simulink model "sampleModel27"  (R2021a)
settings: Solver=VariableStepAuto  StartTime=0.0  StopTime=10.0  RelTol=1e-3
undefined symbols (not defined in the file): DiscIntNeverNeededParam, magnitude, Newton, Raphson
libraries: simulink x49, pid_lib x7
(part 1 of 2)
settings Model: SimulationMode=accelerator  Creator=user  LastModifiedBy=CMelt

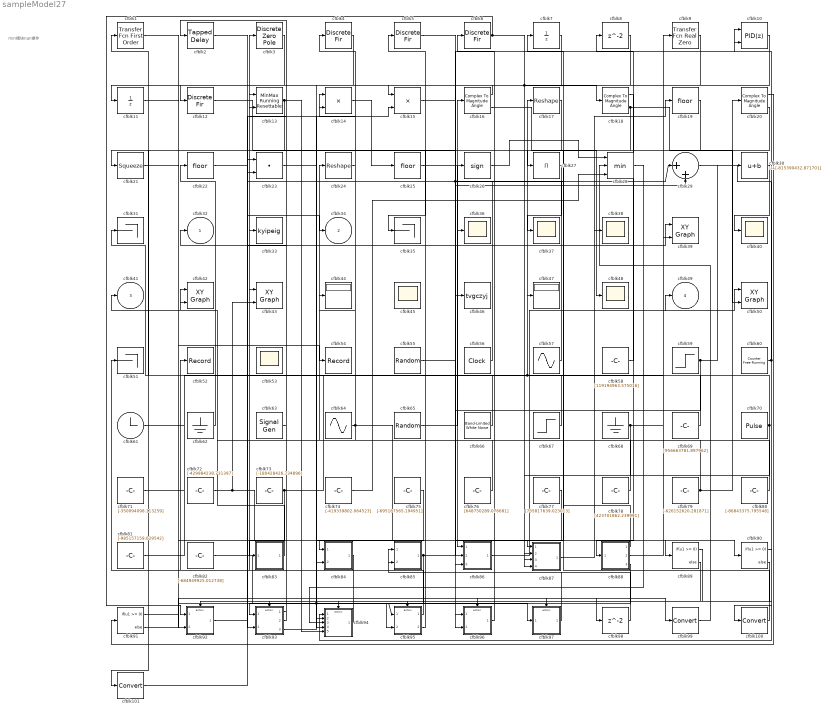
== system sampleModel27 ==
  note: min模块nan操作
  cfblk1 : simulink/Discrete/Transfer Fcn First Order  PoleZ=0.95  ICPrevOutput=0.0  DoSatur=off
  cfblk10 : pid_lib/PID Controller (2DOF)  Controller=PID  Form=Parallel  TimeDomain=Discrete-time  UseExternalTs=off  SampleTime=1  IntegratorMethod=Forward Euler  FilterMethod=Forward Euler  ControllerParametersSource=internal  P=1  I=1  D=0  UseFilter=on  N=100  b=1  c=1  TunerSelectOption=Transfer Function Based (PID Tuner App)  InitialConditionSource=internal  InitialConditionForIntegrator=0  InitialConditionForFilter=0  DifferentiatorICPrevScaledInput=0  ExternalReset=none  TrackingMode=off  Kt=1  LimitOutput=off  SatLimitsSource=internal  UpperSaturationLimit=inf  LowerSaturationLimit=-inf  LinearizeAsGain=off  AntiWindupMode=none  Kb=1  POutMin=[]  POutMax=[]  IOutMin=[]  IOutMax=[]  DOutMin=[]  DOutMax=[]  NOutMin=[]  NOutMax=[]  bOutMin=[]  bOutMax=[]  cOutMin=[]  cOutMax=[]  SumOutMin=[]  SumOutMax=[]  SaturationOutMin=[]  SaturationOutMax=[]  PParamMin=[]  PParamMax=[]  IParamMin=[]  IParamMax=[]  DParamMin=[]  DParamMax=[]  NParamMin=[]  NParamMax=[]  bParamMin=[]  bParamMax=[]  cParamMin=[]  cParamMax=[]  KbParamMin=[]  KbParamMax=[]  KtParamMin=[]  KtParamMax=[]  KbOutMin=[]  KbOutMax=[]  KtOutMin=[]  KtOutMax=[]  IntegratorOutMin=[]  IntegratorOutMax=[]  FilterOutMin=[]  FilterOutMax=[]  SumI1OutMin=[]  SumI1OutMax=[]  SumI2OutMin=[]  SumI2OutMax=[]  SumI3OutMin=[]  SumI3OutMax=[]  SumI4OutMin=[]  SumI4OutMax=[]  SumDOutMin=[]  SumDOutMax=[]  Sum1OutMin=[]  Sum1OutMax=[]  Sum2OutMin=[]  Sum2OutMax=[]  Sum3OutMin=[]  Sum3OutMax=[]  DifferentiatorOutMin=[]  DifferentiatorOutMax=[]  FilterDiffOutCoefMin=[]  FilterDiffOutCoefMax=[]  ReciprocalOutMin=[]  ReciprocalOutMax=[]  SumDenOutMin=[]  SumDenOutMax=[]  SumNumOutMin=[]  SumNumOutMax=[]  DivideOutMin=[]  DivideOutMax=[]  UdiffTsProdOutMin=[]  UdiffTsProdOutMax=[]  NTsProdOutMin=[]  NTsProdOutMax=[]  UintegralTsProdOutMin=[]  UintegralTsProdOutMax=[]  UngainTsProdOutMin=[]  UngainTsProdOutMax=[]  IntegratorContinuousStateAttributes=''  IntegratorStateMustResolveToSignalObject=off  IntegratorRTWStateStorageClass=Auto  FilterContinuousStateAttributes=''  FilterStateMustResolveToSignalObject=off  FilterRTWStateStorageClass=Auto  ParallelPVariant=InternalParameters  IdealPVariant=Disabled  IVariant=InternalParameters  DVariant=InternalParameters  bVariant=InternalParameters  cVariant=InternalParameters  IntegratorVariant=Discrete  SatVariant=Disabled  AWVariant=Passthrough  PCopyVariant=Disabled  TRVariant=Disabled  FdbkBlocksVariant=Forward  IdealPFdbkVariant=Disabled  SatFdbkVariant=Disabled  DerivativeFilterVariant=ForwardEulerFilter  NVariant=InternalParameters  NCopyVariant=Disabled  FilterICVariant=InternalICsFilter  IntegratorICVariant=InternalICs  ExternalResetVariant=Disabled  TRSumVariant=Passthrough  SumFdbkVariant=Disabled  SumVariant=Sum_PID  TsampFilterVariant=InternalTs  TsampNgainVariant=Passthrough  TsampIntegralVariant=Passthrough  ExternalSaturationOutDataTypeStr=Inherit: Same as second input
      settings: SourceProductBaseCode=SL
  cfblk100 : DataTypeConversion
  cfblk101 : DataTypeConversion
  cfblk11 : UnitDelay  HasFrameUpgradeWarning=on
  cfblk{4..6,12} (4 alike) : DiscreteFir  SampleTime=1
  cfblk13 : simulink/Math Operations/MinMax Running Resettable  Function=min  vinit=0.0
  cfblk14 : Product  Inputs=**
  cfblk15 : Product  Inputs=**
  cfblk16 : ComplexToMagnitudeAngle
  cfblk17 : Reshape
  cfblk18 : ComplexToMagnitudeAngle
  cfblk19 : Rounding
  cfblk2 : simulink/Discrete/Tapped Delay  vinit=0.0  samptime=-1  NumDelays=1  DelayOrder=Oldest  includeCurrent=off
  cfblk20 : ComplexToMagnitudeAngle
  cfblk21 : Squeeze
  cfblk22 : Rounding
  cfblk23 : DotProduct  InputSameDT=on  OutDataTypeStr=Inherit: Inherit via internal rule
  cfblk24 : Reshape
  cfblk25 : Rounding
  cfblk26 : Signum
  cfblk27 : Product  Inputs=*
  cfblk28 : MinMax  Inputs=3
  cfblk29 : Sum  Inputs=|++
  cfblk3 : DiscreteZeroPole  Poles=[0 0.5]  Gain=1
  cfblk30 : Bias  Bias=[-815390432.871701]
  cfblk31 : Terminator
  cfblk33 : ToWorkspace  VariableName=kyipeig  SaveFormat=Timeseries  SampleTime=-1
  cfblk35 : Terminator
  cfblk{36..38,40,45,48,53} (7 alike) : Scope
      cfblk45 settings: Floating=on
      cfblk53 settings: Floating=on
  cfblk{39,42..43,50} (4 alike) : simulink/Sinks/XY Graph  xmin=-1  xmax=1  ymin=-1  ymax=1  st=-1
  cfblk44 : Display
  cfblk46 : ToWorkspace  VariableName=tvgczyj  SaveFormat=Timeseries  SampleTime=-1
  cfblk47 : Display
  cfblk51 : Terminator
  cfblk52 : Record  FileSettingsInternal="{\"entries\":[{\"content\":{\"excelSettings\":{\"content\":{},\"type\":\"Streamout.ExcelSettings\"}},\"type\":\"Streamout.FileSettingStorage\",\"uuid\":\"fb11f80e-34bd-4155-aeb7-01b810d6d789\"}],\"packageUris\":[\"http://schema.mathworks.com/mf0/streamout_blocks/R2020a\"],\"version\":\"1.0\"}"  SignalsInternal="{\"entries\":[{\"content\":{\"signals\":[{\"content\":{\"blockPath\":[\"sampleModel27/cfblk52\"],\"channel\":[],\"dimensions\":[1],\"domain\":\"samplemodel27/cfblk52\",\"lineColor\":\"#a2142f\",\"plots\":[1],\"port\":1,\"sid\":[\"\"],\"signalID\":891,\"signalName\":\"cfblk84\"},\"type\":\"RecordBlkView.Signal\",\"uuid\":\"6f85a095-4475-43d3-bab9-3dbcc0fecad7\"}]},\"type\":\"RecordBlkView.InputSignals\",\"uuid\":\"24e3b0c2-4f19-493b-93a7-05a205e117ae\"}],\"packageUris\":[\"http://schema.mathworks.com/mf0/streamout_blocks/R2020a\"],\"version\":\"1.0\"}"  VisualizationBindings="{\"sparklinesplugin\":{\"info\":[{\"bindingParametersList\":[],\"subplotID\":1}]}}"
  cfblk54 : Record  FileSettingsInternal="{\"entries\":[{\"content\":{\"excelSettings\":{\"content\":{},\"type\":\"Streamout.ExcelSettings\"}},\"type\":\"Streamout.FileSettingStorage\",\"uuid\":\"661a3fc6-d036-46d0-a4c7-a8be5b92de13\"}],\"packageUris\":[\"http://schema.mathworks.com/mf0/streamout_blocks/R2020a\"],\"version\":\"1.0\"}"  SignalsInternal="{\"entries\":[{\"content\":{\"signals\":[{\"content\":{\"blockPath\":[\"sampleModel27/cfblk54\"],\"channel\":[],\"dimensions\":[1],\"domain\":\"samplemodel27/cfblk54\",\"lineColor\":\"#139fff\",\"plots\":[1],\"port\":1,\"sid\":[\"\"],\"signalID\":895,\"signalName\":\"cfblk21\"},\"type\":\"RecordBlkView.Signal\",\"uuid\":\"1e160afe-88b1-4798-9b6e-19891c68b1a2\"}]},\"type\":\"RecordBlkView.InputSignals\",\"uuid\":\"bd873b34-5c71-4cc0-af38-2544e9a0ace2\"}],\"packageUris\":[\"http://schema.mathworks.com/mf0/streamout_blocks/R2020a\"],\"version\":\"1.0\"}"  VisualizationBindings="{\"sparklinesplugin\":{\"info\":[{\"bindingParametersList\":[],\"subplotID\":1}]}}"
  cfblk55 : RandomNumber  Mean=[-1249.450853]  Variance=[75448.037597]  Seed=[754077994.000000]  SampleTime=0.1
  cfblk56 : DigitalClock
  cfblk57 : Sin  Amplitude=[-963722435.247906]  Bias=[930160760.058033]  SampleTime=0
  cfblk58 : Constant  Value=[119194963.575016]  SampleTime=1
  cfblk59 : Step  Time=[33.000000]  Before=[-955328328.233696]  After=[-779935419.294909]  SampleTime=0
  cfblk60 : simulink/Sources/Counter Free-Running  NumBits=[42.000000]  tsamp=-1
  cfblk61 : Clock
  cfblk62 : Ground
  cfblk63 : SignalGenerator  WaveForm=sawtooth  Amplitude=[910247910.621120]  Units=rad/sec
  cfblk64 : Sin  Amplitude=[-129917709.975789]  Bias=[-276116717.461174]  SampleTime=0
  cfblk65 : UniformRandomNumber  Minimum=[-3659398183.640169]  Maximum=[7187088124.881099]  Seed=[85361646.000000]  SampleTime=0.1
  cfblk66 : simulink/Sources/Band-Limited White Noise  Cov=[7101691506.405921]  Ts=0.1  seed=[513787139.000000]
  cfblk67 : Step  Time=[17.000000]  Before=[136149007.270913]  After=[-603107143.045370]  SampleTime=0
  cfblk68 : Ground
  cfblk69 : Constant  Value=[956663781.897962]  SampleTime=1
  cfblk7 : UnitDelay  HasFrameUpgradeWarning=on
  cfblk70 : DiscretePulseGenerator  PulseType=Time based  Amplitude=[-722737795.690040]  Period=[17925385.343940]  PulseWidth=5  PhaseDelay=[6.000000]
  cfblk71 : Constant  Value=[-350094098.113259]  SampleTime=1
  cfblk72 : Constant  Value=[-429984238.731397]  SampleTime=1
  cfblk73 : Constant  Value=[-180428426.734896]  SampleTime=1
  cfblk74 : Constant  Value=[-419339802.064523]  SampleTime=1
  cfblk75 : Constant  Value=[-695187565.194951]  SampleTime=1
  cfblk76 : Constant  Value=[648750289.076681]  SampleTime=1
  cfblk77 : Constant  Value=[735817639.023013]  SampleTime=1
  cfblk78 : Constant  Value=[423701862.239991]  SampleTime=1
  cfblk79 : Constant  Value=[-626152620.281871]  SampleTime=1
  cfblk8 : Delay  SampleTime=1
  cfblk80 : Constant  Value=[-86843375.795548]  SampleTime=1
  cfblk81 : Constant  Value=[-985157159.629542]  SampleTime=1
  cfblk82 : Constant  Value=[-684949925.012738]  SampleTime=1
  cfblk83 : Subsystem
  cfblk84 : Subsystem
  cfblk85 : Subsystem
  cfblk86 : Subsystem
  cfblk87 : Subsystem
  cfblk88 : Subsystem
  cfblk89 : If  IfExpression=u1 >= 0  SampleTime=1
  cfblk9 : simulink/Discrete/Transfer Fcn Real Zero  ZeroZ=0.75  ICPrevInput=0.0  DoSatur=off
      settings: SourceProductBaseCode=SL
  cfblk90 : If  IfExpression=u1 >= 0  SampleTime=1
  cfblk91 : If  IfExpression=u1 >= 0  SampleTime=1
  cfblk92 : Subsystem  TreatAsAtomicUnit=on
  cfblk93 : Subsystem  TreatAsAtomicUnit=on
  cfblk94 : Subsystem  TreatAsAtomicUnit=on
  cfblk95 : Subsystem  TreatAsAtomicUnit=on
  cfblk96 : Subsystem  TreatAsAtomicUnit=on
  cfblk97 : Subsystem  TreatAsAtomicUnit=on
  cfblk98 : Delay  SampleTime=1
  cfblk99 : DataTypeConversion
  cfblk32 : Outport
  cfblk34 : Outport  Port=2
  cfblk41 : Outport  Port=3
  cfblk49 : Outport  Port=4
  wires:
  cfblk3/1 -> cfblk11/1
  cfblk56/1 -> cfblk2/1
  cfblk57/1 -> cfblk6/1
  cfblk65/1 -> cfblk16/1
  cfblk72/1 -> cfblk89/1, cfblk43/2
  cfblk84/1(cfblk2) -> cfblk52/1
  cfblk6/1 -> cfblk92/1(cfblk1), cfblk18/1
  cfblk61/1 -> cfblk17/1
  cfblk94/1(cfblk2) -> cfblk3/1
  cfblk76/1 -> cfblk24/1
  cfblk64/1 -> cfblk14/1, cfblk90/1
  cfblk97/1(cfblk2) -> cfblk85/1(cfblk1)
  cfblk25/1 -> cfblk86/1(cfblk1)
  cfblk60/1 -> cfblk10/1, cfblk100/1
  cfblk19/1 -> cfblk27/1
  cfblk88/1(cfblk2) -> cfblk7/1
  cfblk22/1 -> cfblk14/2
  cfblk86/1(cfblk2) -> cfblk49/1
  cfblk70/1 -> cfblk36/1, cfblk87/2(cfblk11)
  cfblk55/1 -> cfblk96/1(cfblk1)
  cfblk96/1(cfblk2) -> cfblk26/1
  cfblk10/1 -> cfblk86/2(cfblk9), cfblk87/4(cfblk13)
  cfblk16/1 -> cfblk15/1
  cfblk62/1 -> cfblk41/1
  cfblk88/2(cfblk9) -> cfblk50/1
  cfblk16/2 -> cfblk48/1
  cfblk85/1(cfblk2) -> cfblk29/1, cfblk10/2, cfblk95/2(cfblk13)
  cfblk2/1 -> cfblk34/1
  cfblk4/1 -> cfblk92/2(cfblk11)
  cfblk29/1 -> cfblk94/1(cfblk1)
  cfblk26/1 -> cfblk28/1
  cfblk67/1 -> cfblk1/1
  cfblk1/1 -> cfblk97/1(cfblk1)
  cfblk63/1 -> cfblk13/1
  cfblk66/1 -> cfblk22/1
  cfblk71/1 -> cfblk9/1
  cfblk14/1 -> cfblk25/1
  cfblk21/1 -> cfblk54/1
  cfblk24/1 -> cfblk4/1
  cfblk95/1(cfblk2) -> cfblk51/1
  cfblk12/1 -> cfblk46/1
  cfblk81/1 -> cfblk33/1
  cfblk17/1 -> cfblk35/1
  cfblk18/1 -> cfblk88/1(cfblk1)
  cfblk88/3(cfblk10) -> cfblk93/1(cfblk1)
  cfblk77/1 -> cfblk96/2(cfblk7)
  cfblk75/1 -> cfblk94/2(cfblk13)
  cfblk9/1 -> cfblk12/1
  cfblk83/1(cfblk2) -> cfblk42/1
  cfblk95/2(cfblk14) -> cfblk5/1
  cfblk80/1 -> cfblk44/1
  cfblk7/1 -> cfblk93/2(cfblk13)
  cfblk11/1 -> cfblk84/1(cfblk1)
  cfblk58/1 -> cfblk8/1
  cfblk18/2 -> cfblk50/2, cfblk87/1(cfblk1)
  cfblk27/1 -> cfblk37/1
  cfblk69/1 -> cfblk47/1, cfblk31/1
  cfblk15/1 -> cfblk29/2
  cfblk8/1 -> cfblk84/2(cfblk9)
  cfblk82/1 -> cfblk95/1(cfblk1), cfblk94/4(cfblk15)
  cfblk13/1 -> cfblk94/5(cfblk16), cfblk101/1
  cfblk30/1 -> cfblk40/1
  cfblk20/1 -> cfblk91/1
  cfblk28/1 -> cfblk94/3(cfblk14)
  cfblk73/1 -> cfblk38/1, cfblk83/1(cfblk1)
  cfblk79/1 -> cfblk20/1, cfblk42/2
  cfblk93/1(cfblk2) -> cfblk13/2
  cfblk20/2 -> cfblk21/1
  cfblk92/1(cfblk2) -> cfblk39/1
  cfblk59/1 -> cfblk86/3(cfblk10), cfblk30/1
  cfblk93/2(cfblk14) -> cfblk32/1
  cfblk68/1 -> cfblk39/2, cfblk87/3(cfblk12)
  cfblk74/1 -> cfblk28/3
  cfblk78/1 -> cfblk43/1
  cfblk93/3(cfblk15) -> cfblk15/2
  cfblk87/1(cfblk2) -> cfblk19/1
  cfblk89/1 -> cfblk92/Action
  cfblk89/2 -> cfblk93/Action
  cfblk90/1 -> cfblk94/Action
  cfblk90/2 -> cfblk95/Action
  cfblk91/1 -> cfblk96/Action
  cfblk91/2 -> cfblk97/Action
  cfblk5/1 -> cfblk98/1
  cfblk98/1 -> cfblk85/2(cfblk14)
  cfblk23/1 -> cfblk99/1
  cfblk99/1 -> cfblk28/2
  cfblk100/1 -> cfblk23/1
  cfblk101/1 -> cfblk23/2

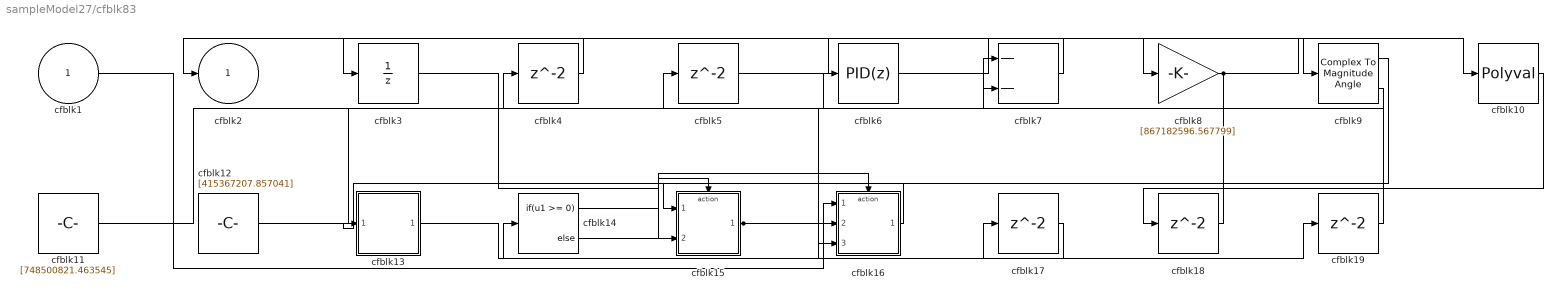
== system sampleModel27/cfblk83 ==
  cfblk1 : Inport
  cfblk10 : Polyval  Coefs=[ +2.081618890e-019, -1.441693666e-014, +4.719686976e-010, -8.536869453e-006, +1.621573104e-001, -8.087801117e+001 ]
  cfblk11 : Constant  Value=[748500821.463545]  SampleTime=1
  cfblk12 : Constant  Value=[415367207.857041]  SampleTime=1
  cfblk13 : Subsystem
  cfblk14 : If  IfExpression=u1 >= 0  SampleTime=1
  cfblk15 : Subsystem  TreatAsAtomicUnit=on
  cfblk16 : Subsystem  TreatAsAtomicUnit=on
  cfblk{4..5,17..19} (5 alike) : Delay  SampleTime=1
  cfblk3 : UnitDelay  HasFrameUpgradeWarning=on
  cfblk6 : pid_lib/PID Controller  Controller=PID  Form=Parallel  TimeDomain=Discrete-time  UseExternalTs=off  SampleTime=1  IntegratorMethod=Forward Euler  FilterMethod=Forward Euler  ControllerParametersSource=internal  P=1  I=1  D=0  UseFilter=on  N=100  TunerSelectOption=Transfer Function Based (PID Tuner App)  InitialConditionSource=internal  InitialConditionForIntegrator=0  InitialConditionForFilter=0  DifferentiatorICPrevScaledInput=0  ExternalReset=none  TrackingMode=off  Kt=1  LimitOutput=off  SatLimitsSource=internal  UpperSaturationLimit=inf  LowerSaturationLimit=-inf  LinearizeAsGain=off  AntiWindupMode=none  Kb=1  POutMin=[]  POutMax=[]  IOutMin=[]  IOutMax=[]  DOutMin=[]  DOutMax=[]  NOutMin=[]  NOutMax=[]  SumOutMin=[]  SumOutMax=[]  SaturationOutMin=[]  SaturationOutMax=[]  PParamMin=[]  PParamMax=[]  IParamMin=[]  IParamMax=[]  DParamMin=[]  DParamMax=[]  NParamMin=[]  NParamMax=[]  KbParamMin=[]  KbParamMax=[]  KtParamMin=[]  KtParamMax=[]  KbOutMin=[]  KbOutMax=[]  KtOutMin=[]  KtOutMax=[]  IntegratorOutMin=[]  IntegratorOutMax=[]  FilterOutMin=[]  FilterOutMax=[]  SumI1OutMin=[]  SumI1OutMax=[]  SumI2OutMin=[]  SumI2OutMax=[]  SumI3OutMin=[]  SumI3OutMax=[]  SumI4OutMin=[]  SumI4OutMax=[]  SumDOutMin=[]  SumDOutMax=[]  DifferentiatorOutMin=[]  DifferentiatorOutMax=[]  FilterDiffOutCoefMin=[]  FilterDiffOutCoefMax=[]  ReciprocalOutMin=[]  ReciprocalOutMax=[]  SumDenOutMin=[]  SumDenOutMax=[]  SumNumOutMin=[]  SumNumOutMax=[]  DivideOutMin=[]  DivideOutMax=[]  UdiffTsProdOutMin=[]  UdiffTsProdOutMax=[]  NTsProdOutMin=[]  NTsProdOutMax=[]  UintegralTsProdOutMin=[]  UintegralTsProdOutMax=[]  UngainTsProdOutMin=[]  UngainTsProdOutMax=[]  IntegratorContinuousStateAttributes=''  IntegratorStateMustResolveToSignalObject=off  IntegratorRTWStateStorageClass=Auto  FilterContinuousStateAttributes=''  FilterStateMustResolveToSignalObject=off  FilterRTWStateStorageClass=Auto  ParallelPVariant=InternalParameters  IdealPVariant=Disabled  IVariant=InternalParameters  DVariant=InternalParameters  IntegratorVariant=Discrete  SatVariant=Disabled  AWVariant=Passthrough  PCopyVariant=Disabled  TRVariant=Disabled  FdbkBlocksVariant=Forward  IdealPFdbkVariant=Disabled  SatFdbkVariant=Disabled  DerivativeFilterVariant=ForwardEulerFilter  NVariant=InternalParameters  NCopyVariant=Disabled  FilterICVariant=InternalICsFilter  IntegratorICVariant=InternalICs  ExternalResetVariant=Disabled  TRSumVariant=Passthrough  SumFdbkVariant=Disabled  SumVariant=Sum_PID  TsampFilterVariant=InternalTs  TsampNgainVariant=Passthrough  TsampIntegralVariant=Passthrough  ExternalSaturationOutDataTypeStr=Inherit: Same as second input
  cfblk7 : Sum  Inputs=--
  cfblk8 : Gain  Gain=[867182596.567799]
  cfblk9 : ComplexToMagnitudeAngle
  cfblk2 : Outport
  wires:
  cfblk7/1 -> cfblk2/1
  cfblk12/1 -> cfblk4/1
  cfblk4/1 -> cfblk3/1
  cfblk15/1(cfblk2) -> cfblk7/2, cfblk17/1
  cfblk1/1 -> cfblk16/1(cfblk1)
  cfblk9/1 -> cfblk13/1(cfblk1)
  cfblk5/1 -> cfblk8/1
  cfblk6/1 -> cfblk9/1
  cfblk16/1(cfblk2) -> cfblk15/1(cfblk1)
  cfblk8/1 -> cfblk10/1, cfblk16/3(cfblk12)
  cfblk3/1 -> cfblk15/2(cfblk16)
  cfblk9/2 -> cfblk16/2(cfblk11)
  cfblk11/1 -> cfblk7/1
  cfblk14/1 -> cfblk15/Action
  cfblk14/2 -> cfblk16/Action
  cfblk17/1 -> cfblk14/1
  cfblk10/1 -> cfblk18/1
  cfblk18/1 -> cfblk5/1
  cfblk13/1(cfblk2) -> cfblk19/1
  cfblk19/1 -> cfblk6/1

== system sampleModel27/cfblk84 ==
  cfblk1 : Inport
  cfblk9 : Inport  Port=2
  cfblk3 : pid_lib/PID Controller  Controller=PID  Form=Parallel  TimeDomain=Discrete-time  UseExternalTs=off  SampleTime=1  IntegratorMethod=Forward Euler  FilterMethod=Forward Euler  ControllerParametersSource=internal  P=1  I=1  D=0  UseFilter=on  N=100  TunerSelectOption=Transfer Function Based (PID Tuner App)  InitialConditionSource=internal  InitialConditionForIntegrator=0  InitialConditionForFilter=0  DifferentiatorICPrevScaledInput=0  ExternalReset=none  TrackingMode=off  Kt=1  LimitOutput=off  SatLimitsSource=internal  UpperSaturationLimit=inf  LowerSaturationLimit=-inf  LinearizeAsGain=off  AntiWindupMode=none  Kb=1  POutMin=[]  POutMax=[]  IOutMin=[]  IOutMax=[]  DOutMin=[]  DOutMax=[]  NOutMin=[]  NOutMax=[]  SumOutMin=[]  SumOutMax=[]  SaturationOutMin=[]  SaturationOutMax=[]  PParamMin=[]  PParamMax=[]  IParamMin=[]  IParamMax=[]  DParamMin=[]  DParamMax=[]  NParamMin=[]  NParamMax=[]  KbParamMin=[]  KbParamMax=[]  KtParamMin=[]  KtParamMax=[]  KbOutMin=[]  KbOutMax=[]  KtOutMin=[]  KtOutMax=[]  IntegratorOutMin=[]  IntegratorOutMax=[]  FilterOutMin=[]  FilterOutMax=[]  SumI1OutMin=[]  SumI1OutMax=[]  SumI2OutMin=[]  SumI2OutMax=[]  SumI3OutMin=[]  SumI3OutMax=[]  SumI4OutMin=[]  SumI4OutMax=[]  SumDOutMin=[]  SumDOutMax=[]  DifferentiatorOutMin=[]  DifferentiatorOutMax=[]  FilterDiffOutCoefMin=[]  FilterDiffOutCoefMax=[]  ReciprocalOutMin=[]  ReciprocalOutMax=[]  SumDenOutMin=[]  SumDenOutMax=[]  SumNumOutMin=[]  SumNumOutMax=[]  DivideOutMin=[]  DivideOutMax=[]  UdiffTsProdOutMin=[]  UdiffTsProdOutMax=[]  NTsProdOutMin=[]  NTsProdOutMax=[]  UintegralTsProdOutMin=[]  UintegralTsProdOutMax=[]  UngainTsProdOutMin=[]  UngainTsProdOutMax=[]  IntegratorContinuousStateAttributes=''  IntegratorStateMustResolveToSignalObject=off  IntegratorRTWStateStorageClass=Auto  FilterContinuousStateAttributes=''  FilterStateMustResolveToSignalObject=off  FilterRTWStateStorageClass=Auto  ParallelPVariant=InternalParameters  IdealPVariant=Disabled  IVariant=InternalParameters  DVariant=InternalParameters  IntegratorVariant=Discrete  SatVariant=Disabled  AWVariant=Passthrough  PCopyVariant=Disabled  TRVariant=Disabled  FdbkBlocksVariant=Forward  IdealPFdbkVariant=Disabled  SatFdbkVariant=Disabled  DerivativeFilterVariant=ForwardEulerFilter  NVariant=InternalParameters  NCopyVariant=Disabled  FilterICVariant=InternalICsFilter  IntegratorICVariant=InternalICs  ExternalResetVariant=Disabled  TRSumVariant=Passthrough  SumFdbkVariant=Disabled  SumVariant=Sum_PID  TsampFilterVariant=InternalTs  TsampNgainVariant=Passthrough  TsampIntegralVariant=Passthrough  ExternalSaturationOutDataTypeStr=Inherit: Same as second input
  cfblk4 : DiscreteIntegrator  ICPrevOutput=DiscIntNeverNeededParam  ICPrevScaledInput=DiscIntNeverNeededParam
  cfblk5 : Constant  Value=[435902225.259876]  SampleTime=1
  cfblk6 : Constant  Value=[507414533.863744]  SampleTime=1
  cfblk7 : Constant  Value=[-778207180.895854]  SampleTime=1
  cfblk8 : Subsystem
  cfblk2 : Outport
  wires:
  cfblk9/1 -> cfblk8/1(cfblk1)
  cfblk5/1 -> cfblk2/1
  cfblk7/1 -> cfblk8/2(cfblk11)
  cfblk6/1 -> cfblk3/1
  cfblk1/1 -> cfblk8/3(cfblk12)
  cfblk3/1 -> cfblk8/4(cfblk13)
  cfblk8/1(cfblk2) -> cfblk4/1

== system sampleModel27/cfblk85 ==
  cfblk1 : Inport
  cfblk14 : Inport  Port=2
  cfblk10 : Constant  Value=[-748821143.501719]  SampleTime=1
  cfblk11 : Constant  Value=[-142338457.475266]  SampleTime=1
  cfblk12 : Constant  Value=[-157921268.774217]  SampleTime=1
  cfblk13 : Subsystem
  cfblk3 : DiscreteFilter  SampleTime=1
  cfblk4 : DiscreteTransferFcn  SampleTime=1
  cfblk5 : DiscreteFilter  SampleTime=1
  cfblk6 : Sum
  cfblk7 : simulink/Math Operations/Slider Gain  gain=1  low=0  high=2
  cfblk8 : Reshape
  cfblk9 : Reshape
  cfblk2 : Outport
  wires:
  cfblk10/1 -> cfblk4/1
  cfblk8/1 -> cfblk7/1
  cfblk14/1 -> cfblk8/1
  cfblk4/1 -> cfblk3/1
  cfblk11/1 -> cfblk6/1
  cfblk1/1 -> cfblk6/2
  cfblk7/1 -> cfblk2/1
  cfblk3/1 -> cfblk9/1
  cfblk9/1 -> cfblk13/1(cfblk1)
  cfblk6/1 -> cfblk5/1

== system sampleModel27/cfblk86 ==
  cfblk1 : Inport
  cfblk9 : Inport  Port=2
  cfblk10 : Inport  Port=3
  cfblk3 : DiscreteFilter  SampleTime=1
  cfblk4 : Sin  TimeSource=Use external signal  SampleTime=0
  cfblk5 : Math  Operator=log  SaturateOnIntegerOverflow=on
  cfblk6 : Sum  Inputs=+
  cfblk7 : Product
  cfblk8 : Constant  Value=[232564695.069627]  SampleTime=1
  cfblk2 : Outport
  wires:
  cfblk8/1 -> cfblk6/1
  cfblk3/1 -> cfblk7/1
  cfblk6/1 -> cfblk7/2
  cfblk1/1 -> cfblk3/1
  cfblk5/1 -> cfblk2/1
  cfblk10/1 -> cfblk5/1
  cfblk7/1 -> cfblk4/1

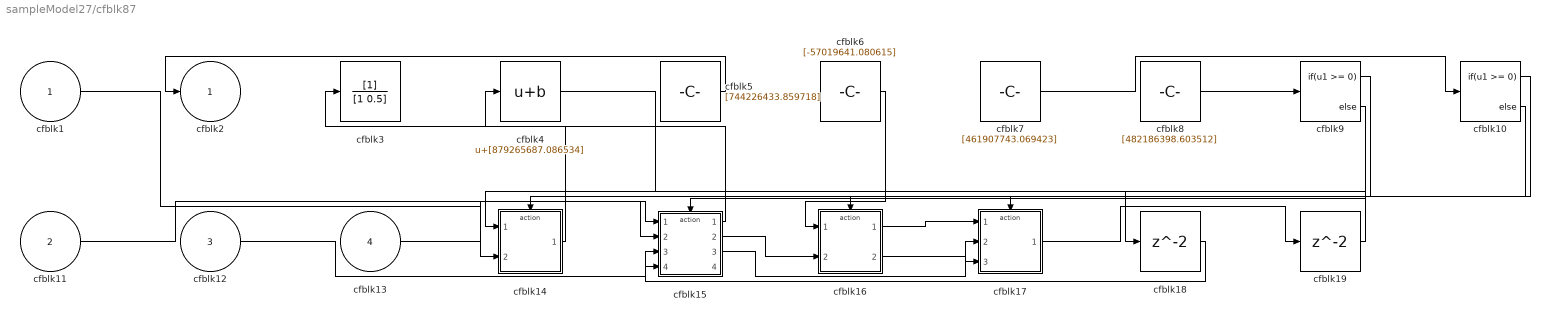
== system sampleModel27/cfblk87 ==
  cfblk1 : Inport
  cfblk11 : Inport  Port=2
  cfblk12 : Inport  Port=3
  cfblk13 : Inport  Port=4
  cfblk10 : If  IfExpression=u1 >= 0  SampleTime=1
  cfblk14 : Subsystem  TreatAsAtomicUnit=on
  cfblk15 : Subsystem  TreatAsAtomicUnit=on
  cfblk16 : Subsystem  TreatAsAtomicUnit=on
  cfblk17 : Subsystem  TreatAsAtomicUnit=on
  cfblk18 : Delay  SampleTime=1
  cfblk19 : Delay  SampleTime=1
  cfblk3 : DiscreteFilter  SampleTime=1
  cfblk4 : Bias  Bias=[879265687.086534]
  cfblk5 : Constant  Value=[744226433.859718]  SampleTime=1
  cfblk6 : Constant  Value=[-57019641.080615]  SampleTime=1
  cfblk7 : Constant  Value=[461907743.069423]  SampleTime=1
  cfblk8 : Constant  Value=[482186398.603512]  SampleTime=1
  cfblk9 : If  IfExpression=u1 >= 0  SampleTime=1
  cfblk2 : Outport
  wires:
  cfblk11/1 -> cfblk15/1(cfblk1)
  cfblk7/1 -> cfblk10/1
  cfblk5/1 -> cfblk2/1
  cfblk14/1(cfblk2) -> cfblk4/1
  cfblk8/1 -> cfblk9/1
  cfblk15/1(cfblk2) -> cfblk3/1
  cfblk6/1 -> cfblk16/1(cfblk1)
  cfblk1/1 -> cfblk14/2(cfblk14)
  cfblk15/2(cfblk15) -> cfblk16/2(cfblk9)
  cfblk16/1(cfblk2) -> cfblk17/1(cfblk1)
  cfblk15/3(cfblk16) -> cfblk17/2(cfblk6)
  cfblk13/1 -> cfblk15/2(cfblk12)
  cfblk16/2(cfblk10) -> cfblk17/3(cfblk7)
  cfblk12/1 -> cfblk15/3(cfblk13)
  cfblk9/1 -> cfblk14/Action
  cfblk9/2 -> cfblk15/Action
  cfblk10/1 -> cfblk16/Action
  cfblk10/2 -> cfblk17/Action
  cfblk4/1 -> cfblk18/1
  cfblk18/1 -> cfblk15/4(cfblk14)
  cfblk17/1(cfblk2) -> cfblk19/1
  cfblk19/1 -> cfblk14/1(cfblk1)

== system sampleModel27/cfblk88 ==
  cfblk1 : Inport
  cfblk11 : Subsystem  TreatAsAtomicUnit=on
  cfblk12 : Subsystem  TreatAsAtomicUnit=on
  cfblk13 : Delay  SampleTime=1
  cfblk3 : UnitDelay  HasFrameUpgradeWarning=on
  cfblk4 : Sum  Inputs=+
  cfblk5 : Constant  Value=[997414698.843862]  SampleTime=1
  cfblk6 : Constant  Value=[-297248467.896038]  SampleTime=1
  cfblk7 : Constant  Value=[156034469.193004]  SampleTime=1
  cfblk8 : If  IfExpression=u1 >= 0  SampleTime=1
  cfblk2 : Outport
  cfblk9 : Outport  Port=2
  cfblk10 : Outport  Port=3
  wires:
  cfblk1/1 -> cfblk10/1
  cfblk7/1 -> cfblk4/1
  cfblk6/1 -> cfblk12/1(cfblk1), cfblk12/4(cfblk12)
  cfblk12/1(cfblk2) -> cfblk2/1, cfblk13/1
  cfblk5/1 -> cfblk3/1, cfblk12/3(cfblk11)
  cfblk4/1 -> cfblk11/1(cfblk1), cfblk9/1
  cfblk3/1 -> cfblk11/2(cfblk7)
  cfblk11/1(cfblk2) -> cfblk12/2(cfblk10)
  cfblk8/1 -> cfblk11/Action
  cfblk8/2 -> cfblk12/Action
  cfblk13/1 -> cfblk8/1

== system sampleModel27/cfblk92 ==
  cfblk1 : Inport
  cfblk11 : Inport  Port=2
  Action Port : ActionPort  ActionPortLabel=if(u1 >= 0)
  cfblk10 : Subsystem
  cfblk12 : Delay
  cfblk3 : pid_lib/PID Controller  Controller=PID  Form=Parallel  TimeDomain=Discrete-time  UseExternalTs=off  SampleTime=-1  IntegratorMethod=Forward Euler  FilterMethod=Forward Euler  ControllerParametersSource=internal  P=1  I=1  D=0  UseFilter=on  N=100  TunerSelectOption=Transfer Function Based (PID Tuner App)  InitialConditionSource=internal  InitialConditionForIntegrator=0  InitialConditionForFilter=0  DifferentiatorICPrevScaledInput=0  ExternalReset=none  TrackingMode=off  Kt=1  LimitOutput=off  SatLimitsSource=internal  UpperSaturationLimit=inf  LowerSaturationLimit=-inf  LinearizeAsGain=off  AntiWindupMode=none  Kb=1  POutMin=[]  POutMax=[]  IOutMin=[]  IOutMax=[]  DOutMin=[]  DOutMax=[]  NOutMin=[]  NOutMax=[]  SumOutMin=[]  SumOutMax=[]  SaturationOutMin=[]  SaturationOutMax=[]  PParamMin=[]  PParamMax=[]  IParamMin=[]  IParamMax=[]  DParamMin=[]  DParamMax=[]  NParamMin=[]  NParamMax=[]  KbParamMin=[]  KbParamMax=[]  KtParamMin=[]  KtParamMax=[]  KbOutMin=[]  KbOutMax=[]  KtOutMin=[]  KtOutMax=[]  IntegratorOutMin=[]  IntegratorOutMax=[]  FilterOutMin=[]  FilterOutMax=[]  SumI1OutMin=[]  SumI1OutMax=[]  SumI2OutMin=[]  SumI2OutMax=[]  SumI3OutMin=[]  SumI3OutMax=[]  SumI4OutMin=[]  SumI4OutMax=[]  SumDOutMin=[]  SumDOutMax=[]  DifferentiatorOutMin=[]  DifferentiatorOutMax=[]  FilterDiffOutCoefMin=[]  FilterDiffOutCoefMax=[]  ReciprocalOutMin=[]  ReciprocalOutMax=[]  SumDenOutMin=[]  SumDenOutMax=[]  SumNumOutMin=[]  SumNumOutMax=[]  DivideOutMin=[]  DivideOutMax=[]  UdiffTsProdOutMin=[]  UdiffTsProdOutMax=[]  NTsProdOutMin=[]  NTsProdOutMax=[]  UintegralTsProdOutMin=[]  UintegralTsProdOutMax=[]  UngainTsProdOutMin=[]  UngainTsProdOutMax=[]  IntegratorContinuousStateAttributes=''  IntegratorStateMustResolveToSignalObject=off  IntegratorRTWStateStorageClass=Auto  FilterContinuousStateAttributes=''  FilterStateMustResolveToSignalObject=off  FilterRTWStateStorageClass=Auto  ParallelPVariant=InternalParameters  IdealPVariant=Disabled  IVariant=InternalParameters  DVariant=InternalParameters  IntegratorVariant=Discrete  SatVariant=Disabled  AWVariant=Passthrough  PCopyVariant=Disabled  TRVariant=Disabled  FdbkBlocksVariant=Forward  IdealPFdbkVariant=Disabled  SatFdbkVariant=Disabled  DerivativeFilterVariant=ForwardEulerFilter  NVariant=InternalParameters  NCopyVariant=Disabled  FilterICVariant=InternalICsFilter  IntegratorICVariant=InternalICs  ExternalResetVariant=Disabled  TRSumVariant=Passthrough  SumFdbkVariant=Disabled  SumVariant=Sum_PID  TsampFilterVariant=InternalTs  TsampNgainVariant=Passthrough  TsampIntegralVariant=Passthrough  ExternalSaturationOutDataTypeStr=Inherit: Same as second input
  cfblk4 : Reshape
  cfblk5 : Sin  TimeSource=Use external signal  SampleTime=0
  cfblk6 : DotProduct  InputSameDT=on  OutDataTypeStr=Inherit: Inherit via internal rule
  cfblk7 : Assignment  DiagnosticForDimensions=Warning  IndexOptions=Index vector (dialog)  Indices=1  OutputSizes=1
  cfblk8 : Constant  Value=[683401835.628090]  SampleTime=1
  cfblk9 : Constant  Value=[104221195.868824]  SampleTime=1
  cfblk2 : Outport
  wires:
  cfblk10/1(cfblk2) -> cfblk4/1
  cfblk1/1 -> cfblk3/1
  cfblk3/1 -> cfblk7/1
  cfblk5/1 -> cfblk2/1
  cfblk9/1 -> cfblk7/2
  cfblk11/1 -> cfblk5/1
  cfblk7/1 -> cfblk6/2
  cfblk8/1 -> cfblk10/1(cfblk1)
  cfblk6/1 -> cfblk10/2(cfblk10)
  cfblk4/1 -> cfblk12/1
  cfblk12/1 -> cfblk6/1

== system sampleModel27/cfblk93 ==
  cfblk1 : Inport
  cfblk13 : Inport  Port=2
  Action Port : ActionPort  ActionPortLabel=else
  cfblk10 : Constant  Value=[573308680.084131]  SampleTime=1
  cfblk11 : Subsystem
  cfblk12 : Subsystem
  cfblk3 : Sqrt  Operator=rSqrt  AlgorithmType=Newton-Raphson  SaturateOnIntegerOverflow=on
  cfblk4 : Squeeze
  cfblk5 : Constant  Value=[768949352.583149]  SampleTime=1
  cfblk6 : Constant  Value=[915452941.264737]  SampleTime=1
  cfblk7 : Constant  Value=[-433515266.185090]  SampleTime=1
  cfblk8 : Constant  Value=[-269447240.998842]  SampleTime=1
  cfblk9 : Constant  Value=[16042384.070648]  SampleTime=1
  cfblk2 : Outport
  cfblk14 : Outport  Port=2
  cfblk15 : Outport  Port=3
  wires:
  cfblk1/1 -> cfblk14/1
  cfblk6/1 -> cfblk2/1
  cfblk8/1 -> cfblk15/1
  cfblk7/1 -> cfblk12/1(cfblk1)
  cfblk13/1 -> cfblk12/2(cfblk7)
  cfblk3/1 -> cfblk4/1
  cfblk5/1 -> cfblk11/1(cfblk1)
  cfblk12/1(cfblk2) -> cfblk11/2(cfblk16)
  cfblk11/1(cfblk2) -> cfblk3/1
  cfblk9/1 -> cfblk11/3(cfblk17)

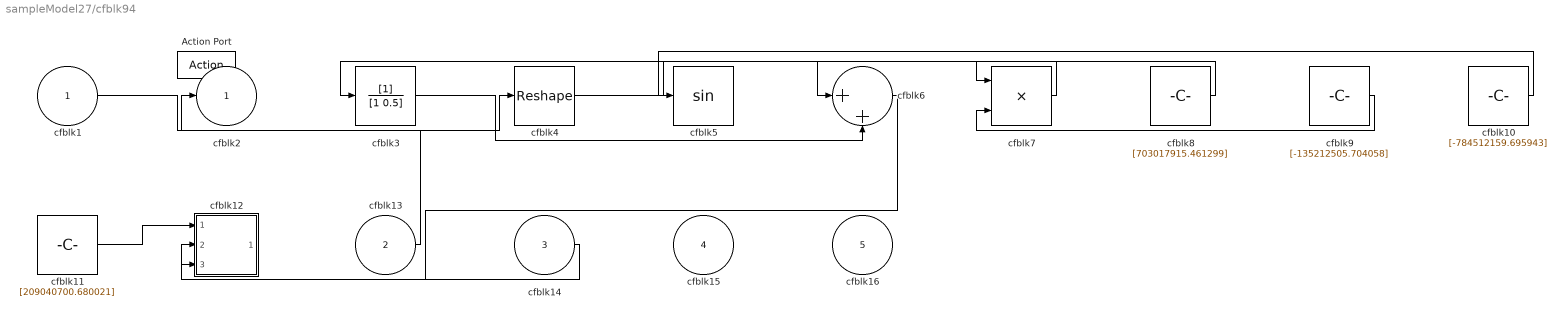
== system sampleModel27/cfblk94 ==
  cfblk1 : Inport
  cfblk13 : Inport  Port=2
  cfblk14 : Inport  Port=3
  cfblk15 : Inport  Port=4
  cfblk16 : Inport  Port=5
  Action Port : ActionPort  ActionPortLabel=if(u1 >= 0)
  cfblk10 : Constant  Value=[-784512159.695943]  SampleTime=1
  cfblk11 : Constant  Value=[209040700.680021]  SampleTime=1
  cfblk12 : Subsystem
  cfblk3 : DiscreteFilter
  cfblk4 : Reshape
  cfblk5 : Trigonometry
  cfblk6 : Sum  Inputs=|++
  cfblk7 : Product  Inputs=**
  cfblk8 : Constant  Value=[703017915.461299]  SampleTime=1
  cfblk9 : Constant  Value=[-135212505.704058]  SampleTime=1
  cfblk2 : Outport
  wires:
  cfblk13/1 -> cfblk2/1
  cfblk4/1 -> cfblk7/1
  cfblk9/1 -> cfblk7/2
  cfblk10/1 -> cfblk5/1
  cfblk7/1 -> cfblk3/1
  cfblk1/1 -> cfblk4/1
  cfblk11/1 -> cfblk12/1(cfblk1)
  cfblk6/1 -> cfblk12/2(cfblk9)
  cfblk14/1 -> cfblk12/3(cfblk10)
  cfblk8/1 -> cfblk6/1
  cfblk3/1 -> cfblk6/2

== system sampleModel27/cfblk95 ==
  cfblk1 : Inport
  cfblk13 : Inport  Port=2
  Action Port : ActionPort  ActionPortLabel=else
  cfblk10 : Constant  Value=[-944507749.993055]  SampleTime=1
  cfblk11 : Subsystem
  cfblk12 : Subsystem
  cfblk15 : Delay
  cfblk3 : simulink/Discrete/Tapped Delay  vinit=0.0  samptime=-1  NumDelays=1  DelayOrder=Oldest  includeCurrent=off
  cfblk4 : DiscreteIntegrator  SampleTime=-1  ICPrevOutput=DiscIntNeverNeededParam  ICPrevScaledInput=DiscIntNeverNeededParam
  cfblk5 : Sum  Inputs=+-
  cfblk6 : Sqrt  Operator=rSqrt  AlgorithmType=Newton-Raphson  SaturateOnIntegerOverflow=on
  cfblk7 : Constant  Value=[52912862.636736]  SampleTime=1
  cfblk8 : Constant  Value=[-355964147.219021]  SampleTime=1
  cfblk9 : Constant  Value=[-253451230.848444]  SampleTime=1
  cfblk2 : Outport
  cfblk14 : Outport  Port=2
  wires:
  cfblk10/1 -> cfblk4/1
  cfblk1/1 -> cfblk6/1
  cfblk4/1 -> cfblk11/1(cfblk1)
  cfblk11/1(cfblk2) -> cfblk2/1
  cfblk6/1 -> cfblk12/1(cfblk1)
  cfblk8/1 -> cfblk14/1
  cfblk13/1 -> cfblk5/1
  cfblk9/1 -> cfblk11/2(cfblk9)
  cfblk3/1 -> cfblk5/2
  cfblk12/1(cfblk2) -> cfblk3/1
  cfblk5/1 -> cfblk15/1
  cfblk15/1 -> cfblk12/2(cfblk8)

== system sampleModel27/cfblk96 ==
  cfblk1 : Inport
  cfblk7 : Inport  Port=2
  Action Port : ActionPort  ActionPortLabel=if(u1 >= 0)
  cfblk3 : Sqrt  Operator=rSqrt  AlgorithmType=Newton-Raphson  SaturateOnIntegerOverflow=on
  cfblk4 : Polyval  Coefs=[ +2.081618890e-019, -1.441693666e-014, +4.719686976e-010, -8.536869453e-006, +1.621573104e-001, -8.087801117e+001 ]
  cfblk5 : Product  Inputs=*
  cfblk6 : Constant  Value=[745650532.881739]  SampleTime=1
  cfblk2 : Outport
  wires:
  cfblk3/1 -> cfblk2/1
  cfblk6/1 -> cfblk4/1
  cfblk1/1 -> cfblk5/1
  cfblk5/1 -> cfblk3/1

== system sampleModel27/cfblk97 ==
  cfblk1 : Inport
  Action Port : ActionPort  ActionPortLabel=else
  cfblk3 : simulink/Discrete/Transfer Fcn Lead or Lag  PoleZ=0.95  ZeroZ=0.75  ICPrevOutput=0.0  ICPrevInput=0.0  DoSatur=off
      settings: SourceProductBaseCode=SL
  cfblk4 : Sqrt  Operator=rSqrt  AlgorithmType=Newton-Raphson  SaturateOnIntegerOverflow=on
  cfblk5 : Assignment  DiagnosticForDimensions=Warning  IndexOptions=Index vector (dialog)  Indices=1  OutputSizes=1
  cfblk6 : Constant  Value=[308239103.638663]  SampleTime=1
  cfblk7 : Constant  Value=[184913364.083033]  SampleTime=1
  cfblk8 : Delay
  cfblk2 : Outport
  wires:
  cfblk3/1 -> cfblk5/1
  cfblk5/1 -> cfblk4/1
  cfblk6/1 -> cfblk5/2
  cfblk7/1 -> cfblk2/1
  cfblk4/1 -> cfblk8/1
  cfblk8/1 -> cfblk3/1

== system sampleModel27/cfblk83/cfblk13 ==
  cfblk1 : Inport
  cfblk3 : DiscreteTransferFcn  SampleTime=1
  cfblk4 : pid_lib/PID Controller  Controller=PID  Form=Parallel  TimeDomain=Discrete-time  UseExternalTs=off  SampleTime=1  IntegratorMethod=Forward Euler  FilterMethod=Forward Euler  ControllerParametersSource=internal  P=1  I=1  D=0  UseFilter=on  N=100  TunerSelectOption=Transfer Function Based (PID Tuner App)  InitialConditionSource=internal  InitialConditionForIntegrator=0  InitialConditionForFilter=0  DifferentiatorICPrevScaledInput=0  ExternalReset=none  TrackingMode=off  Kt=1  LimitOutput=off  SatLimitsSource=internal  UpperSaturationLimit=inf  LowerSaturationLimit=-inf  LinearizeAsGain=off  AntiWindupMode=none  Kb=1  POutMin=[]  POutMax=[]  IOutMin=[]  IOutMax=[]  DOutMin=[]  DOutMax=[]  NOutMin=[]  NOutMax=[]  SumOutMin=[]  SumOutMax=[]  SaturationOutMin=[]  SaturationOutMax=[]  PParamMin=[]  PParamMax=[]  IParamMin=[]  IParamMax=[]  DParamMin=[]  DParamMax=[]  NParamMin=[]  NParamMax=[]  KbParamMin=[]  KbParamMax=[]  KtParamMin=[]  KtParamMax=[]  KbOutMin=[]  KbOutMax=[]  KtOutMin=[]  KtOutMax=[]  IntegratorOutMin=[]  IntegratorOutMax=[]  FilterOutMin=[]  FilterOutMax=[]  SumI1OutMin=[]  SumI1OutMax=[]  SumI2OutMin=[]  SumI2OutMax=[]  SumI3OutMin=[]  SumI3OutMax=[]  SumI4OutMin=[]  SumI4OutMax=[]  SumDOutMin=[]  SumDOutMax=[]  DifferentiatorOutMin=[]  DifferentiatorOutMax=[]  FilterDiffOutCoefMin=[]  FilterDiffOutCoefMax=[]  ReciprocalOutMin=[]  ReciprocalOutMax=[]  SumDenOutMin=[]  SumDenOutMax=[]  SumNumOutMin=[]  SumNumOutMax=[]  DivideOutMin=[]  DivideOutMax=[]  UdiffTsProdOutMin=[]  UdiffTsProdOutMax=[]  NTsProdOutMin=[]  NTsProdOutMax=[]  UintegralTsProdOutMin=[]  UintegralTsProdOutMax=[]  UngainTsProdOutMin=[]  UngainTsProdOutMax=[]  IntegratorContinuousStateAttributes=''  IntegratorStateMustResolveToSignalObject=off  IntegratorRTWStateStorageClass=Auto  FilterContinuousStateAttributes=''  FilterStateMustResolveToSignalObject=off  FilterRTWStateStorageClass=Auto  ParallelPVariant=InternalParameters  IdealPVariant=Disabled  IVariant=InternalParameters  DVariant=InternalParameters  IntegratorVariant=Discrete  SatVariant=Disabled  AWVariant=Passthrough  PCopyVariant=Disabled  TRVariant=Disabled  FdbkBlocksVariant=Forward  IdealPFdbkVariant=Disabled  SatFdbkVariant=Disabled  DerivativeFilterVariant=ForwardEulerFilter  NVariant=InternalParameters  NCopyVariant=Disabled  FilterICVariant=InternalICsFilter  IntegratorICVariant=InternalICs  ExternalResetVariant=Disabled  TRSumVariant=Passthrough  SumFdbkVariant=Disabled  SumVariant=Sum_PID  TsampFilterVariant=InternalTs  TsampNgainVariant=Passthrough  TsampIntegralVariant=Passthrough  ExternalSaturationOutDataTypeStr=Inherit: Same as second input
  cfblk5 : simulink/Discrete/Difference  ICPrevInput=0.0  OutMin=[]  OutMax=[]  OutDataTypeStr=Inherit: Inherit via back propagation  OutDataType=fixdt(1, 16)  OutScaling=2^-10  DoSatur=off
  cfblk6 : Constant  Value=[677722872.783128]  SampleTime=1
  cfblk7 : Subsystem
  cfblk8 : Delay  SampleTime=1
  cfblk2 : Outport
  wires:
  cfblk5/1 -> cfblk4/1
  cfblk6/1 -> cfblk2/1
  cfblk1/1 -> cfblk5/1
  cfblk7/1(cfblk2) -> cfblk3/1
  cfblk4/1 -> cfblk7/2(cfblk13)
  cfblk3/1 -> cfblk8/1
  cfblk8/1 -> cfblk7/1(cfblk1)

== system sampleModel27/cfblk83/cfblk15 ==
  cfblk1 : Inport
  cfblk16 : Inport  Port=2
  Action Port : ActionPort  ActionPortLabel=if(u1 >= 0)
  cfblk10 : Constant  Value=[698916418.216047]  SampleTime=1
  cfblk11 : Constant  Value=[645425733.943067]  SampleTime=1
  cfblk12 : Constant  Value=[-917550418.540600]  SampleTime=1
  cfblk13 : Constant  Value=[532379415.671905]  SampleTime=1
  cfblk14 : Subsystem
  cfblk15 : Subsystem
  cfblk3 : DiscreteStateSpace  SampleTime=-1
  cfblk4 : ComplexToMagnitudeAngle
  cfblk5 : Sum  Inputs=+
  cfblk6 : Assignment  DiagnosticForDimensions=Warning  IndexOptions=Index vector (dialog)  Indices=1  OutputSizes=1
  cfblk7 : Constant  Value=[-250469021.620363]  SampleTime=1
  cfblk8 : Constant  Value=[648509559.341775]  SampleTime=1
  cfblk9 : Constant  Value=[243846627.983253]  SampleTime=1
  cfblk2 : Outport
  wires:
  cfblk7/1 -> cfblk4/1
  cfblk15/1(cfblk2) -> cfblk14/1(cfblk1)
  cfblk14/1(cfblk2) -> cfblk5/1
  cfblk14/2(cfblk10) -> cfblk3/1
  cfblk10/1 -> cfblk2/1
  cfblk4/1 -> cfblk6/1
  cfblk12/1 -> cfblk6/2
  cfblk4/2 -> cfblk15/1(cfblk1)
  cfblk8/1 -> cfblk15/2(cfblk9)
  cfblk16/1 -> cfblk15/3(cfblk10)

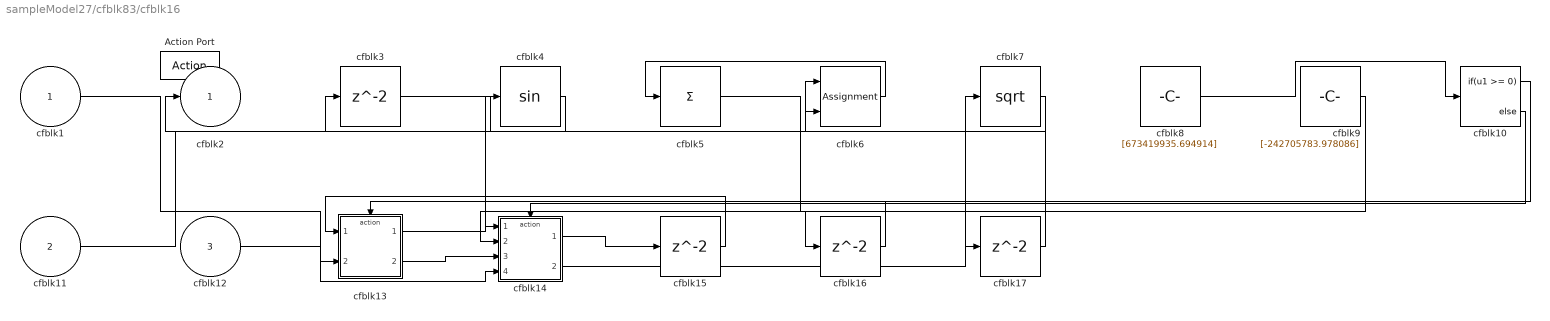
== system sampleModel27/cfblk83/cfblk16 ==
  cfblk1 : Inport
  cfblk11 : Inport  Port=2
  cfblk12 : Inport  Port=3
  Action Port : ActionPort  ActionPortLabel=else
  cfblk10 : If  IfExpression=u1 >= 0  SampleTime=1
  cfblk13 : Subsystem  TreatAsAtomicUnit=on
  cfblk14 : Subsystem  TreatAsAtomicUnit=on
  cfblk{3,15..17} (4 alike) : Delay
  cfblk4 : Trigonometry
  cfblk5 : Sum  Inputs=+
  cfblk6 : Assignment  DiagnosticForDimensions=Warning  IndexOptions=Index vector (dialog)  Indices=1  OutputSizes=1
  cfblk7 : Sqrt  SaturateOnIntegerOverflow=on
  cfblk8 : Constant  Value=[673419935.694914]  SampleTime=1
  cfblk9 : Constant  Value=[-242705783.978086]  SampleTime=1
  cfblk2 : Outport
  wires:
  cfblk11/1 -> cfblk6/1
  cfblk8/1 -> cfblk10/1
  cfblk6/1 -> cfblk5/1
  cfblk4/1 -> cfblk2/1
  cfblk3/1 -> cfblk6/2
  cfblk13/1(cfblk2) -> cfblk4/1
  cfblk1/1 -> cfblk13/2(cfblk7)
  cfblk14/2(cfblk11) -> cfblk7/1
  cfblk9/1 -> cfblk14/2(cfblk8)
  cfblk13/2(cfblk8) -> cfblk14/3(cfblk9)
  cfblk12/1 -> cfblk14/4(cfblk10)
  cfblk10/1 -> cfblk13/Action
  cfblk10/2 -> cfblk14/Action
  cfblk14/1(cfblk2) -> cfblk15/1
  cfblk15/1 -> cfblk13/1(cfblk1)
  cfblk7/1 -> cfblk16/1
  cfblk16/1 -> cfblk14/1(cfblk1)
  cfblk5/1 -> cfblk17/1
  cfblk17/1 -> cfblk3/1

== system sampleModel27/cfblk84/cfblk8 ==
  cfblk1 : Inport
  cfblk11 : Inport  Port=2
  cfblk12 : Inport  Port=3
  cfblk13 : Inport  Port=4
  cfblk10 : If  IfExpression=u1 >= 0  SampleTime=1
  cfblk14 : Subsystem  TreatAsAtomicUnit=on
  cfblk15 : Subsystem  TreatAsAtomicUnit=on
  cfblk16 : Delay  SampleTime=1
  cfblk17 : Delay  SampleTime=1
  cfblk3 : DiscreteTransferFcn  SampleTime=1
  cfblk4 : ComplexToMagnitudeAngle
  cfblk5 : Product
  cfblk6 : Sin  TimeSource=Use external signal  SampleTime=0
  cfblk7 : Constant  Value=[-289768238.779738]  SampleTime=1
  cfblk8 : Constant  Value=[27539374.384663]  SampleTime=1
  cfblk9 : Constant  Value=[503948235.286263]  SampleTime=1
  cfblk2 : Outport
  wires:
  cfblk3/1 -> cfblk10/1
  cfblk14/1(cfblk2) -> cfblk5/1
  cfblk9/1 -> cfblk14/1(cfblk1)
  cfblk7/1 -> cfblk6/1
  cfblk1/1 -> cfblk4/1
  cfblk13/1 -> cfblk2/1
  cfblk4/1 -> cfblk15/1(cfblk1)
  cfblk8/1 -> cfblk14/2(cfblk11)
  cfblk14/3(cfblk14) -> cfblk5/2
  cfblk10/1 -> cfblk14/Action
  cfblk10/2 -> cfblk15/Action
  cfblk5/1 -> cfblk16/1
  cfblk16/1 -> cfblk14/3(cfblk12)
  cfblk14/2(cfblk13) -> cfblk17/1
  cfblk17/1 -> cfblk3/1

== system sampleModel27/cfblk85/cfblk13 ==
  cfblk1 : Inport
  cfblk10 : Subsystem
  cfblk3 : simulink/Discrete/Tapped Delay  vinit=0.0  samptime=-1  NumDelays=1  DelayOrder=Oldest  includeCurrent=off
  cfblk4 : Product  Inputs=*
  cfblk5 : Assignment  DiagnosticForDimensions=Warning  IndexOptions=Index vector (dialog)  Indices=1  OutputSizes=1
  cfblk6 : Constant  Value=[371068949.789462]  SampleTime=1
  cfblk7 : Constant  Value=[35481309.384586]  SampleTime=1
  cfblk8 : Constant  Value=[-296335346.825991]  SampleTime=1
  cfblk9 : Constant  Value=[238789030.728096]  SampleTime=1
  cfblk2 : Outport
  wires:
  cfblk10/1(cfblk2) -> cfblk3/1
  cfblk4/1 -> cfblk5/1
  cfblk10/2(cfblk11) -> cfblk5/2
  cfblk6/1 -> cfblk10/1(cfblk1)
  cfblk1/1 -> cfblk4/1
  cfblk7/1 -> cfblk2/1
  cfblk9/1 -> cfblk10/2(cfblk10)

== system sampleModel27/cfblk87/cfblk14 ==
  cfblk1 : Inport
  cfblk14 : Inport  Port=2
  Action Port : ActionPort  ActionPortLabel=if(u1 >= 0)
  cfblk10 : Constant  Value=[412426713.170433]  SampleTime=1
  cfblk11 : Constant  Value=[710028861.377292]  SampleTime=1
  cfblk12 : Constant  Value=[236050670.583528]  SampleTime=1
  cfblk13 : Subsystem
  cfblk15 : Delay
  cfblk3 : simulink/Discrete/Transfer Fcn Real Zero  ZeroZ=0.75  ICPrevInput=0.0  DoSatur=off
      settings: SourceProductBaseCode=SL
  cfblk4 : DotProduct  InputSameDT=on  OutDataTypeStr=Inherit: Inherit via internal rule
  cfblk5 : Sqrt  Operator=rSqrt  AlgorithmType=Newton-Raphson  SaturateOnIntegerOverflow=on
  cfblk6 : PermuteDimensions
  cfblk7 : Assignment  DiagnosticForDimensions=Warning  IndexOptions=Index vector (dialog)  Indices=1  OutputSizes=1
  cfblk8 : ComplexToMagnitudeAngle
  cfblk9 : Constant  Value=[352322347.633126]  SampleTime=1
  cfblk2 : Outport
  wires:
  cfblk5/1 -> cfblk3/1
  cfblk13/1(cfblk2) -> cfblk8/1
  cfblk6/1 -> cfblk5/1
  cfblk13/2(cfblk9) -> cfblk7/1
  cfblk11/1 -> cfblk7/2
  cfblk9/1 -> cfblk6/1
  cfblk12/1 -> cfblk4/1
  cfblk14/1 -> cfblk13/1(cfblk1)
  cfblk1/1 -> cfblk13/2(cfblk6)
  cfblk10/1 -> cfblk4/2
  cfblk7/1 -> cfblk2/1
  cfblk3/1 -> cfblk13/4(cfblk8)
  cfblk8/1 -> cfblk15/1
  cfblk15/1 -> cfblk13/3(cfblk7)

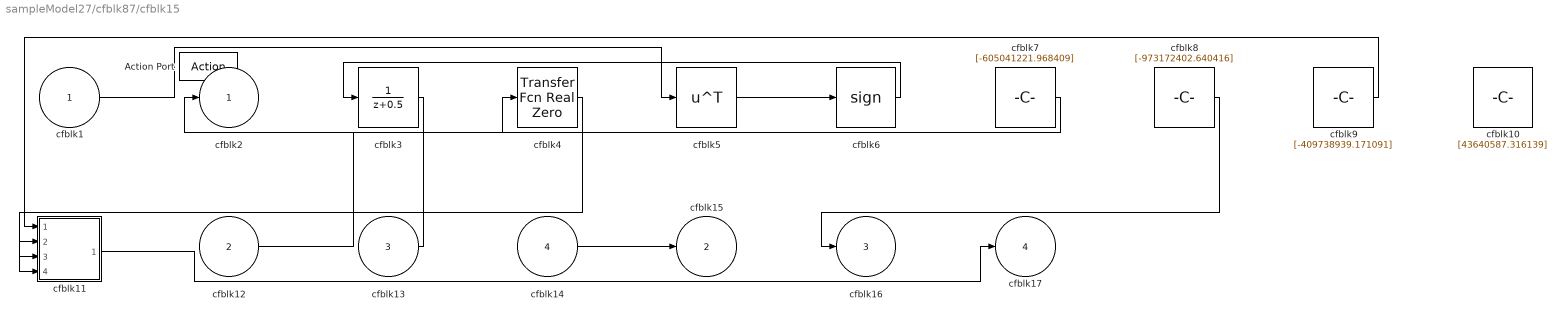
== system sampleModel27/cfblk87/cfblk15 ==
  cfblk1 : Inport
  cfblk12 : Inport  Port=2
  cfblk13 : Inport  Port=3
  cfblk14 : Inport  Port=4
  Action Port : ActionPort  ActionPortLabel=else
  cfblk10 : Constant  Value=[43640587.316139]  SampleTime=1
  cfblk11 : Subsystem
  cfblk3 : DiscreteTransferFcn
  cfblk4 : simulink/Discrete/Transfer Fcn Real Zero  ZeroZ=0.75  ICPrevInput=0.0  DoSatur=off
      settings: SourceProductBaseCode=SL
  cfblk5 : Math  Operator=transpose  SaturateOnIntegerOverflow=on
  cfblk6 : Signum
  cfblk7 : Constant  Value=[-605041221.968409]  SampleTime=1
  cfblk8 : Constant  Value=[-973172402.640416]  SampleTime=1
  cfblk9 : Constant  Value=[-409738939.171091]  SampleTime=1
  cfblk2 : Outport
  cfblk15 : Outport  Port=2
  cfblk16 : Outport  Port=3
  cfblk17 : Outport  Port=4
  wires:
  cfblk7/1 -> cfblk2/1
  cfblk11/1(cfblk2) -> cfblk17/1
  cfblk12/1 -> cfblk4/1
  cfblk14/1 -> cfblk15/1
  cfblk8/1 -> cfblk16/1
  cfblk5/1 -> cfblk6/1
  cfblk1/1 -> cfblk5/1
  cfblk9/1 -> cfblk11/1(cfblk1)
  cfblk6/1 -> cfblk3/1
  cfblk13/1 -> cfblk11/2(cfblk10)
  cfblk3/1 -> cfblk11/3(cfblk11)
  cfblk4/1 -> cfblk11/4(cfblk12)

== system sampleModel27/cfblk87/cfblk16 ==
  cfblk1 : Inport
  cfblk9 : Inport  Port=2
  Action Port : ActionPort  ActionPortLabel=if(u1 >= 0)
  cfblk3 : DiscreteIntegrator  SampleTime=-1  ICPrevOutput=DiscIntNeverNeededParam  ICPrevScaledInput=DiscIntNeverNeededParam
  cfblk4 : Signum
  cfblk5 : Sum  Inputs=+-
  cfblk6 : Constant  Value=[-267441294.667689]  SampleTime=1
  cfblk7 : Constant  Value=[-30377741.992494]  SampleTime=1
  cfblk8 : Constant  Value=[129829913.635514]  SampleTime=1
  cfblk2 : Outport
  cfblk10 : Outport  Port=2
  wires:
  cfblk1/1 -> cfblk3/1
  cfblk7/1 -> cfblk4/1
  cfblk4/1 -> cfblk2/1
  cfblk6/1 -> cfblk10/1
  cfblk3/1 -> cfblk5/1
  cfblk9/1 -> cfblk5/2

== system sampleModel27/cfblk87/cfblk17 ==
  cfblk1 : Inport
  cfblk6 : Inport  Port=2
  cfblk7 : Inport  Port=3
  Action Port : ActionPort  ActionPortLabel=else
  cfblk10 : Delay
  cfblk3 : PermuteDimensions
  cfblk4 : Constant  Value=[510337954.853319]  SampleTime=1
  cfblk5 : If  IfExpression=u1 >= 0  SampleTime=1
  cfblk8 : Subsystem  TreatAsAtomicUnit=on
  cfblk9 : Subsystem  TreatAsAtomicUnit=on
  cfblk2 : Outport
  wires:
  cfblk6/1 -> cfblk8/1(cfblk1), cfblk3/1
  cfblk7/1 -> cfblk9/2(cfblk11), cfblk8/3(cfblk12)
  cfblk4/1 -> cfblk8/2(cfblk11)
  cfblk1/1 -> cfblk9/3(cfblk12), cfblk9/4(cfblk13)
  cfblk3/1 -> cfblk5/1, cfblk8/6(cfblk15)
  cfblk9/1(cfblk2) -> cfblk2/1, cfblk8/4(cfblk13), cfblk8/5(cfblk14)
  cfblk5/1 -> cfblk8/Action
  cfblk5/2 -> cfblk9/Action
  cfblk8/1(cfblk2) -> cfblk10/1
  cfblk10/1 -> cfblk9/1(cfblk1)

== system sampleModel27/cfblk88/cfblk11 ==
  cfblk1 : Inport
  cfblk7 : Inport  Port=2
  Action Port : ActionPort  ActionPortLabel=if(u1 >= 0)
  cfblk3 : DiscreteFilter
  cfblk4 : Constant  Value=[747414045.311086]  SampleTime=1
  cfblk5 : Constant  Value=[-450526849.498372]  SampleTime=1
  cfblk6 : Subsystem
  cfblk2 : Outport
  wires:
  cfblk4/1 -> cfblk3/1
  cfblk5/1 -> cfblk6/1(cfblk1)
  cfblk7/1 -> cfblk6/2(cfblk11)
  cfblk1/1 -> cfblk6/3(cfblk12)
  cfblk6/1(cfblk2) -> cfblk2/1

== system sampleModel27/cfblk88/cfblk12 ==
  cfblk1 : Inport
  cfblk10 : Inport  Port=2
  cfblk11 : Inport  Port=3
  cfblk12 : Inport  Port=4
  Action Port : ActionPort  ActionPortLabel=else
  cfblk3 : DiscreteFir
  cfblk4 : DiscreteTransferFcn
  cfblk5 : simulink/Discrete/Transfer Fcn Real Zero  ZeroZ=0.75  ICPrevInput=0.0  DoSatur=off
      settings: SourceProductBaseCode=SL
  cfblk6 : Sum  Inputs=+
  cfblk7 : Sum  Inputs=|++
  cfblk8 : Constant  Value=[-136610867.233684]  SampleTime=1
  cfblk9 : Constant  Value=[-769176903.204337]  SampleTime=1
  cfblk2 : Outport
  wires:
  cfblk5/1 -> cfblk2/1
  cfblk10/1 -> cfblk4/1
  cfblk6/1 -> cfblk5/1
  cfblk7/1 -> cfblk3/1
  cfblk1/1 -> cfblk7/1
  cfblk12/1 -> cfblk7/2
  cfblk11/1 -> cfblk6/1

== system sampleModel27/cfblk92/cfblk10 ==
  cfblk1 : Inport
  cfblk10 : Inport  Port=2
  cfblk11 : Delay
  cfblk3 : simulink/Discrete/Tapped Delay  vinit=0.0  samptime=-1  NumDelays=1  DelayOrder=Oldest  includeCurrent=off
  cfblk4 : Sum  Inputs=|++
  cfblk5 : Rounding
  cfblk6 : simulink/Math Operations/Slider Gain  gain=1  low=0  high=2
  cfblk7 : Sum  Inputs=|++
  cfblk8 : Constant  Value=[610243995.049341]  SampleTime=1
  cfblk9 : Constant  Value=[451104389.173087]  SampleTime=1
  cfblk2 : Outport
  wires:
  cfblk8/1 -> cfblk4/1
  cfblk6/1 -> cfblk7/1
  cfblk1/1 -> cfblk2/1
  cfblk3/1 -> cfblk6/1
  cfblk9/1 -> cfblk7/2
  cfblk4/1 -> cfblk5/1
  cfblk7/1 -> cfblk4/2
  cfblk5/1 -> cfblk11/1
  cfblk11/1 -> cfblk3/1

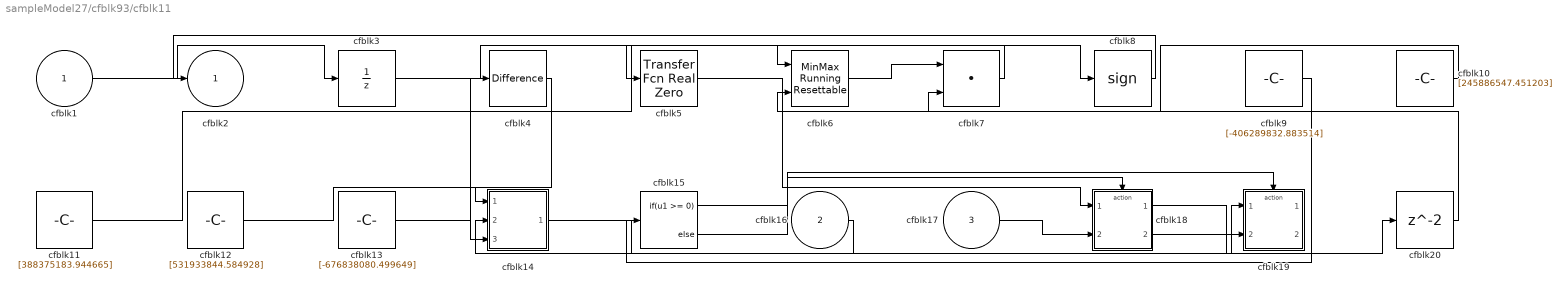
== system sampleModel27/cfblk93/cfblk11 ==
  cfblk1 : Inport
  cfblk16 : Inport  Port=2
  cfblk17 : Inport  Port=3
  cfblk10 : Constant  Value=[245886547.451203]  SampleTime=1
  cfblk11 : Constant  Value=[388375183.944665]  SampleTime=1
  cfblk12 : Constant  Value=[531933844.584928]  SampleTime=1
  cfblk13 : Constant  Value=[-676838080.499649]  SampleTime=1
  cfblk14 : Subsystem
  cfblk15 : If  IfExpression=u1 >= 0  SampleTime=1
  cfblk18 : Subsystem  TreatAsAtomicUnit=on
  cfblk19 : Subsystem  TreatAsAtomicUnit=on
  cfblk20 : Delay
  cfblk3 : UnitDelay  SampleTime=-1  HasFrameUpgradeWarning=on
  cfblk4 : simulink/Discrete/Difference  ICPrevInput=0.0  OutMin=[]  OutMax=[]  OutDataTypeStr=Inherit: Inherit via back propagation  OutDataType=fixdt(1, 16)  OutScaling=2^-10  DoSatur=off
  cfblk5 : simulink/Discrete/Transfer Fcn Real Zero  ZeroZ=0.75  ICPrevInput=0.0  DoSatur=off
      settings: SourceProductBaseCode=SL
  cfblk6 : simulink/Math Operations/MinMax Running Resettable  Function=min  vinit=0.0
  cfblk7 : DotProduct  InputSameDT=on  OutDataTypeStr=Inherit: Inherit via internal rule
  cfblk8 : Signum
  cfblk9 : Constant  Value=[-406289832.883514]  SampleTime=1
  cfblk2 : Outport
  wires:
  cfblk5/1 -> cfblk18/1(cfblk1)
  cfblk6/1 -> cfblk7/1
  cfblk11/1 -> cfblk8/1
  cfblk1/1 -> cfblk3/1
  cfblk7/1 -> cfblk5/1
  cfblk8/1 -> cfblk2/1
  cfblk12/1 -> cfblk14/1(cfblk1)
  cfblk14/1(cfblk2) -> cfblk19/1(cfblk1)
  cfblk17/1 -> cfblk18/2(cfblk11)
  cfblk9/1 -> cfblk15/1
  cfblk18/1(cfblk2) -> cfblk19/2(cfblk9)
  cfblk3/1 -> cfblk6/1
  cfblk10/1 -> cfblk7/2
  cfblk13/1 -> cfblk4/1
  cfblk16/1 -> cfblk14/2(cfblk9)
  cfblk4/1 -> cfblk14/3(cfblk10)
  cfblk15/1 -> cfblk18/Action
  cfblk15/2 -> cfblk19/Action
  cfblk18/2(cfblk12) -> cfblk20/1
  cfblk20/1 -> cfblk6/2

== system sampleModel27/cfblk93/cfblk12 ==
  cfblk1 : Inport
  cfblk7 : Inport  Port=2
  cfblk3 : Math  Operator=hypot  SaturateOnIntegerOverflow=on
  cfblk4 : Sum  Inputs=|++
  cfblk5 : Sin  TimeSource=Use external signal  SampleTime=0
  cfblk6 : Subsystem
  cfblk8 : Delay
  cfblk2 : Outport
  wires:
  cfblk1/1 -> cfblk4/1, cfblk3/2
  cfblk3/1 -> cfblk6/1(cfblk1)
  cfblk7/1 -> cfblk5/1
  cfblk5/1 -> cfblk6/2(cfblk6)
  cfblk4/1 -> cfblk2/1
  cfblk6/1(cfblk2) -> cfblk4/2
  cfblk6/2(cfblk7) -> cfblk8/1
  cfblk8/1 -> cfblk3/1

== system sampleModel27/cfblk94/cfblk12 ==
  cfblk1 : Inport
  cfblk9 : Inport  Port=2
  cfblk10 : Inport  Port=3
  cfblk3 : simulink/Discrete/Transfer Fcn Real Zero  ZeroZ=0.75  ICPrevInput=0.0  DoSatur=off
      settings: SourceProductBaseCode=SL
  cfblk4 : Abs
  cfblk5 : MinMax  Function=max  Inputs=2
  cfblk6 : Trigonometry
  cfblk7 : Math  Operator=magnitude^2  SaturateOnIntegerOverflow=on
  cfblk8 : Constant  Value=[-553503809.206278]  SampleTime=1
  cfblk2 : Outport
  wires:
  cfblk7/1 -> cfblk6/1
  cfblk8/1 -> cfblk3/1
  cfblk1/1 -> cfblk5/1
  cfblk4/1 -> cfblk2/1
  cfblk9/1 -> cfblk7/1
  cfblk10/1 -> cfblk5/2
  cfblk3/1 -> cfblk4/1

== system sampleModel27/cfblk95/cfblk11 ==
  cfblk1 : Inport
  cfblk9 : Inport  Port=2
  cfblk3 : Sqrt  SaturateOnIntegerOverflow=on
  cfblk4 : ComplexToRealImag
  cfblk5 : Squeeze
  cfblk6 : Constant  Value=[330928315.236022]  SampleTime=1
  cfblk7 : Constant  Value=[-227215950.451623]  SampleTime=1
  cfblk8 : Constant  Value=[452675836.354420]  SampleTime=1
  cfblk2 : Outport
  cfblk10 : Outport  Port=2
  wires:
  cfblk7/1 -> cfblk2/1
  cfblk4/1 -> cfblk5/1
  cfblk8/1 -> cfblk4/1
  cfblk9/1 -> cfblk3/1
  cfblk6/1 -> cfblk10/1

== system sampleModel27/cfblk95/cfblk12 ==
  cfblk1 : Inport
  cfblk8 : Inport  Port=2
  cfblk10 : Subsystem  TreatAsAtomicUnit=on
  cfblk11 : Subsystem  TreatAsAtomicUnit=on
  cfblk3 : Bias  Bias=[-132026990.166725]
  cfblk4 : UnaryMinus
  cfblk5 : Constant  Value=[-835599937.577167]  SampleTime=1
  cfblk6 : Constant  Value=[-95187884.059846]  SampleTime=1
  cfblk7 : If  IfExpression=u1 >= 0  SampleTime=1
  cfblk2 : Outport
  cfblk9 : Outport  Port=2
  wires:
  cfblk11/1(cfblk2) -> cfblk10/1(cfblk1)
  cfblk3/1 -> cfblk7/1, cfblk11/3(cfblk13)
  cfblk6/1 -> cfblk3/1, cfblk11/4(cfblk14)
  cfblk5/1 -> cfblk4/1
  cfblk4/1 -> cfblk2/1, cfblk10/3(cfblk8)
  cfblk10/1(cfblk2) -> cfblk9/1
  cfblk8/1 -> cfblk11/1(cfblk1), cfblk11/5(cfblk15)
  cfblk1/1 -> cfblk11/2(cfblk12)
  cfblk11/2(cfblk16) -> cfblk10/2(cfblk7)
  cfblk7/1 -> cfblk10/Action
  cfblk7/2 -> cfblk11/Action
